simulink model "Design2simulink"  (R2023b)
settings: Solver=VariableStepAuto  StartTime=0.0  StopTime=2000  RelTol=1e-3
libraries: slpidlib x1, simulink x1
settings Model: Creator=anbos17  LastModifiedBy=dame9
settings RTWCC: GPUComputeCapability=5.0

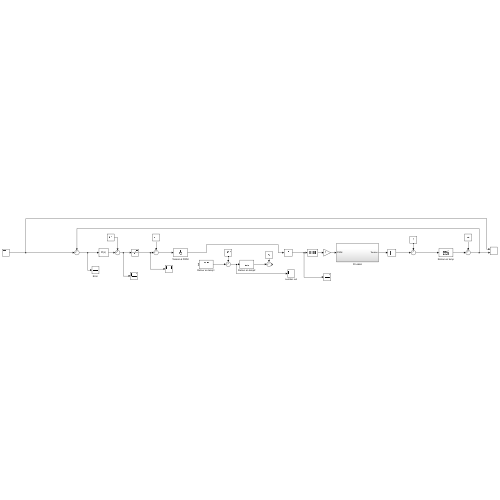
[thumbnail: Simulink's stored preview of the top-level diagram]
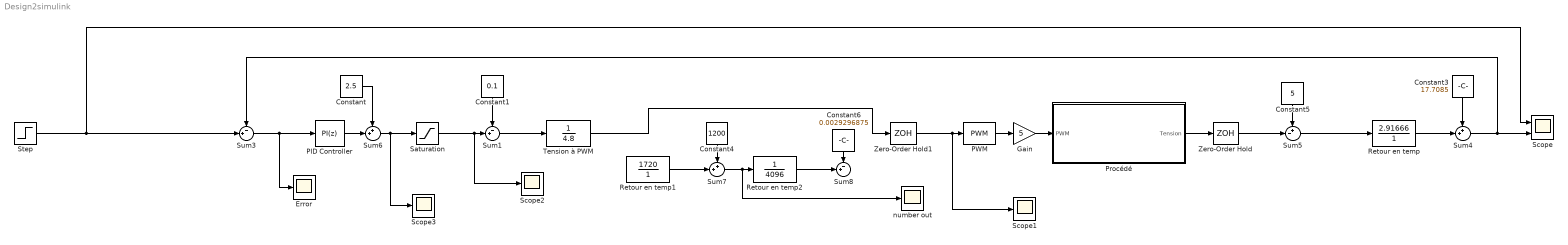
== system Design2simulink ==
  Constant : Constant  Value=2.5
  Constant1 : Constant  Value=0.1
  Constant3 : Constant  Value=17.7085
  Constant4 : Constant  Value=1200
  Constant5 : Constant  Value=5
  Constant6 : Constant  Value=0.0029296875
  Error : Scope
  Gain : Gain  Gain=5
  PID Controller : slpidlib/PID Controller  Controller=PI  Form=Parallel  TimeDomain=Discrete-time  UseExternalTs=off  SampleTime=1  IntegratorMethod=Forward Euler  FilterMethod=Forward Euler  ControllerParametersSource=internal  P=163.93/(50 * 6.34)  I=0.005  UseKiTs=off  D=0.1  N=100  UseFilter=on  TunerSelectOption=Transfer Function Based (PID Tuner App)  InitialConditionSource=internal  InitialConditionForIntegrator=0  InitialConditionForFilter=0  DifferentiatorICPrevScaledInput=0  ExternalReset=none  TrackingMode=off  Kt=1  LimitOutput=off  SatLimitsSource=internal  UpperSaturationLimit=inf  LowerSaturationLimit=-inf  LinearizeAsGain=on  AntiWindupMode=none  Kb=1  LimitIntegrator=off  UpperIntegratorSaturationLimit=inf  LowerIntegratorSaturationLimit=-inf  POutMin=[]  POutMax=[]  IOutMin=[]  IOutMax=[]  DOutMin=[]  DOutMax=[]  NOutMin=[]  NOutMax=[]  SumOutMin=[]  SumOutMax=[]  SaturationOutMin=[]  SaturationOutMax=[]  PParamMin=[]  PParamMax=[]  IParamMin=[]  IParamMax=[]  DParamMin=[]  DParamMax=[]  NParamMin=[]  NParamMax=[]  KbParamMin=[]  KbParamMax=[]  KtParamMin=[]  KtParamMax=[]  KbOutMin=[]  KbOutMax=[]  KtOutMin=[]  KtOutMax=[]  IntegratorOutMin=[]  IntegratorOutMax=[]  FilterOutMin=[]  FilterOutMax=[]  SumI1OutMin=[]  SumI1OutMax=[]  SumI2OutMin=[]  SumI2OutMax=[]  SumI3OutMin=[]  SumI3OutMax=[]  SumI4OutMin=[]  SumI4OutMax=[]  SumDOutMin=[]  SumDOutMax=[]  DifferentiatorOutMin=[]  DifferentiatorOutMax=[]  FilterDiffOutCoefMin=[]  FilterDiffOutCoefMax=[]  ReciprocalOutMin=[]  ReciprocalOutMax=[]  SumDenOutMin=[]  SumDenOutMax=[]  SumNumOutMin=[]  SumNumOutMax=[]  DivideOutMin=[]  DivideOutMax=[]  UdiffTsProdOutMin=[]  UdiffTsProdOutMax=[]  NTsProdOutMin=[]  NTsProdOutMax=[]  UintegralTsProdOutMin=[]  UintegralTsProdOutMax=[]  UngainTsProdOutMin=[]  UngainTsProdOutMax=[]  ClampingZeroOutDataTypeStr=Inherit: Inherit via back propagation  ClampingZeroOutMin=[]  ClampingZeroOutMax=[]  FilterDenConstantOutDataTypeStr=Inherit: Inherit via back propagation  FilterDenConstantOutMin=[]  FilterDenConstantOutMax=[]  PCopyOutDataTypeStr=Inherit: Inherit via back propagation  PCopyOutMin=[]  PCopyOutMax=[]  NCopyOutDataTypeStr=Inherit: Inherit via back propagation  NCopyOutMin=[]  NCopyOutMax=[]  IntegratorContinuousStateAttributes=''  IntegratorStateMustResolveToSignalObject=off  IntegratorRTWStateStorageClass=Auto  FilterContinuousStateAttributes=''  FilterStateMustResolveToSignalObject=off  FilterRTWStateStorageClass=Auto  ParallelPVariant=InternalParameters  IdealPVariant=Disabled  IVariant=InternalParameters  DVariant=Disabled  IntegratorVariant=Discrete  SatVariant=Disabled  AWVariant=Passthrough  PCopyVariant=Disabled  TRVariant=Disabled  FdbkBlocksVariant=Forward  IdealPFdbkVariant=Disabled  SatFdbkVariant=Disabled  DerivativeFilterVariant=Disabled  NVariant=Disabled  NCopyVariant=Disabled_SignalSpec  FilterICVariant=Disabled  IntegratorICVariant=InternalICs  ExternalResetVariant=Disabled  TRSumVariant=Passthrough  SumFdbkVariant=Disabled  SumVariant=Sum_PI  TsampFilterVariant=InternalTs  TsampNgainVariant=Passthrough  TsampIntegralVariant=Disabled_SignalSpec  ExternalSaturationOutDataTypeStr=Inherit: Same as second input
  PWM : simulink/Discontinuities/PWM  DisableCoverage=on  Period=0.002048  InitialDelay=0  DisallowZeroDutyCycle=off  RunAtFixedTimeIntervals=off  SampleTime=0.1
  Procédé : Subsystem
  Retour en temp : TransferFcn  Numerator=[2.91666]  Denominator=[1]
  Retour en temp1 : TransferFcn  Numerator=[1720]  Denominator=[1]
  Retour en temp2 : TransferFcn  Denominator=[4096]
  Saturation : Saturate  UpperLimit=4.9  LowerLimit=0.1
  Scope : Scope  NumInputPorts=2
  Scope1 : Scope
  Scope2 : Scope
  Scope3 : Scope
  Step : Step  Time=500  Before=25  After=24  SampleTime=0
  Sum1 : Sum  Inputs=-+|  InputSameDT=on  SaturateOnIntegerOverflow=on  OutDataTypeStr=Inherit: Same as first input
  Sum3 : Sum  Inputs=-+|  InputSameDT=on  SaturateOnIntegerOverflow=on  OutDataTypeStr=Inherit: Same as first input
  Sum4 : Sum  Inputs=++|  InputSameDT=on  SaturateOnIntegerOverflow=on  OutDataTypeStr=Inherit: Same as first input
  Sum5 : Sum  Inputs=+-|  InputSameDT=on  SaturateOnIntegerOverflow=on  OutDataTypeStr=Inherit: Same as first input
  Sum6 : Sum  Inputs=++|  InputSameDT=on  SaturateOnIntegerOverflow=on  OutDataTypeStr=Inherit: Same as first input
  Sum7 : Sum  Inputs=++|  InputSameDT=on  SaturateOnIntegerOverflow=on  OutDataTypeStr=Inherit: Same as first input
  Sum8 : Sum  Inputs=-+|  InputSameDT=on  SaturateOnIntegerOverflow=on  OutDataTypeStr=Inherit: Same as first input
  Tension à PWM : TransferFcn  Denominator=[4.8]
  Zero-Order Hold : ZeroOrderHold
  Zero-Order Hold1 : ZeroOrderHold
  number out : Scope
  wires:
  Procédé/1(Tension) -> Zero-Order Hold/1
  Zero-Order Hold/1 -> Sum5/2
  Zero-Order Hold1/1 -> Scope1/1, PWM/1
  Step/1 -> Sum3/2, Scope/1
  Sum4/1 -> Sum3/1, Scope/2
  Retour en temp/1 -> Sum4/2
  Constant3/1 -> Sum4/1
  PWM/1 -> Gain/1
  Gain/1 -> Procédé/1(PWM)
  Constant5/1 -> Sum5/1
  Sum5/1 -> Retour en temp/1
  Sum3/1 -> PID Controller/1, Error/1
  Sum6/1 -> Scope3/1, Saturation/1
  Constant/1 -> Sum6/1
  Constant1/1 -> Sum1/1
  Saturation/1 -> Scope2/1, Sum1/2
  Sum1/1 -> Tension à PWM/1
  Retour en temp1/1 -> Sum7/2
  Constant4/1 -> Sum7/1
  Sum7/1 -> Retour en temp2/1, number out/1
  Constant6/1 -> Sum8/1
  Retour en temp2/1 -> Sum8/2
  PID Controller/1 -> Sum6/2
  Tension à PWM/1 -> Zero-Order Hold1/1

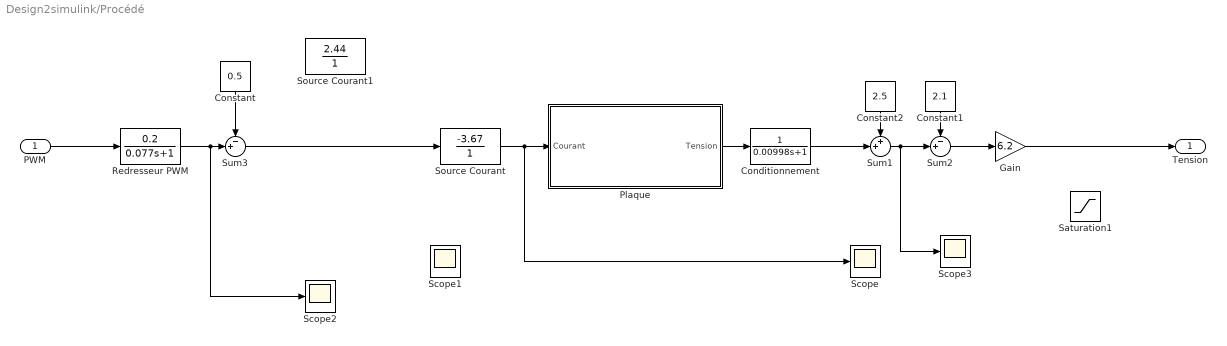
== system Design2simulink/Procédé ==
  PWM : Inport
  Conditionnement : TransferFcn  Denominator=[0.00998 1]
  Constant : Constant  Value=0.5
  Constant1 : Constant  Value=2.1
  Constant2 : Constant  Value=2.5
  Gain : Gain  Gain=6.2
  Plaque : Subsystem
  Redresseur PWM : TransferFcn  Numerator=[0.2]  Denominator=[0.077 1]
  Saturation1 : Saturate  UpperLimit=4.9  LowerLimit=0.1
  Scope{,1..3} (4 alike) : Scope
  Source Courant : TransferFcn  Numerator=[-3.67]  Denominator=[1]
  Source Courant1 : TransferFcn  Numerator=[2.44]  Denominator=[1]
  Sum1 : Sum  Inputs=++|  InputSameDT=on  SaturateOnIntegerOverflow=on  OutDataTypeStr=Inherit: Same as first input
  Sum2 : Sum  Inputs=-+|  InputSameDT=on  SaturateOnIntegerOverflow=on  OutDataTypeStr=Inherit: Same as first input
  Sum3 : Sum  Inputs=-+|  InputSameDT=on  SaturateOnIntegerOverflow=on  OutDataTypeStr=Inherit: Same as first input
  Tension : Outport
  wires:
  Sum1/1 -> Sum2/2, Scope3/1
  Constant2/1 -> Sum1/1
  Plaque/1(Tension) -> Conditionnement/1
  Constant1/1 -> Sum2/1
  Constant/1 -> Sum3/1
  Source Courant/1 -> Scope/1, Plaque/1(Courant)
  Redresseur PWM/1 -> Scope2/1, Sum3/2
  Conditionnement/1 -> Sum1/2
  PWM/1 -> Redresseur PWM/1
  Sum3/1 -> Source Courant/1
  Sum2/1 -> Gain/1
  Gain/1 -> Tension/1

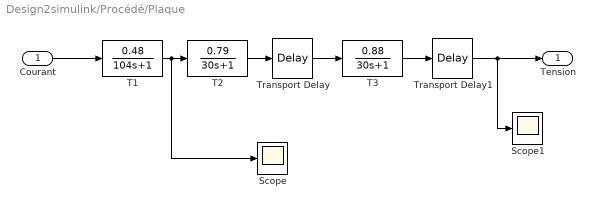
== system Design2simulink/Procédé/Plaque ==
  Courant : Inport
  Scope : Scope
  Scope1 : Scope
  T1 : TransferFcn  Numerator=[0.48]  Denominator=[104 1]
  T2 : TransferFcn  Numerator=[0.79]  Denominator=[30 1]
  T3 : TransferFcn  Numerator=[0.88]  Denominator=[30 1]
  Transport Delay : TransportDelay  DelayTime=4
  Transport Delay1 : TransportDelay  DelayTime=2
  Tension : Outport
  wires:
  Transport Delay/1 -> T3/1
  T1/1 -> Scope/1, T2/1
  T2/1 -> Transport Delay/1
  T3/1 -> Transport Delay1/1
  Courant/1 -> T1/1
  Transport Delay1/1 -> Scope1/1, Tension/1
